simulink model "Test_Case"  (R2017b)
settings: Solver=VariableStepAuto  StartTime=0.0  StopTime=5  RelTol=1e-3
libraries: DigitalControlLib x3
settings Model: Creator=alexandersoussan  LastModifiedBy=alexandersoussan

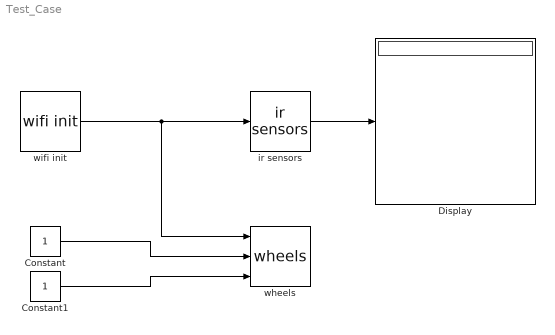
== system Test_Case ==
  Constant : Constant
  Constant1 : Constant
  Display : Display
  ir sensors : DigitalControlLib/ir sensors
  wheels : DigitalControlLib/wheels
  wifi init : DigitalControlLib/wifi init
  wires:
  Constant1/1 -> wheels/3
  Constant/1 -> wheels/2
  wifi init/1 -> wheels/1, ir sensors/1
  ir sensors/1 -> Display/1
